simulink model "SSB_10"  (R2018a)
settings: Solver=VariableStepAuto  StartTime=0.0  StopTime=10.0  MaxStep=0.001  RelTol=1e-3
undefined symbols (not defined in the file or in its folder): magnitude
libraries: dspstat3 x2, dsparch4 x1, commrandsrc3 x1, commanapbnd3 x1
settings Model: Creator=sdf  LastModifiedBy=sdf

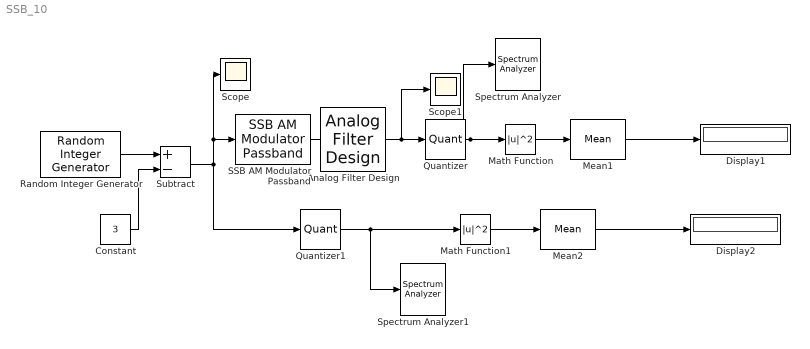
== system SSB_10 ==
  Analog Filter Design : dsparch4/Analog Filter Design  method=Butterworth  filttype=Lowpass  N=8  Wlo=2*pi*300  Whi=80  Rp=2  Rs=40
  Constant : Constant  Value=3
  Display1 : Display
  Display2 : Display
  Math Function : Math  Operator=magnitude^2  SaturateOnIntegerOverflow=on
  Math Function1 : Math  Operator=magnitude^2  SaturateOnIntegerOverflow=on
  Mean1 : dspstat3/Mean  run=on  InputProcessing=Columns as channels (frame based)  reset_popup=None  directionMode=Each column  dimension=1  roiEnable=off  roiType=Rectangles  roiPortion=Entire ROI  roiOutput=Individual statistics for each ROI  roiFlag=off  roundingMode=Floor  overflowMode=off  outputDataTypeStr=Inherit: Same as accumulator  outputMin=[]  outputMax=[]  outputLastDataTypeStr=Inherit: Same as accumulator
  Mean2 : dspstat3/Mean  run=on  InputProcessing=Columns as channels (frame based)  reset_popup=None  directionMode=Each column  dimension=1  roiEnable=off  roiType=Rectangles  roiPortion=Entire ROI  roiOutput=Individual statistics for each ROI  roiFlag=off  roundingMode=Floor  overflowMode=off  outputDataTypeStr=Inherit: Same as accumulator  outputMin=[]  outputMax=[]  outputLastDataTypeStr=Inherit: Same as accumulator
  Quantizer : Quantizer  QuantizationInterval=0.001  LinearizeAsGain=off
  Quantizer1 : Quantizer  QuantizationInterval=0.001  LinearizeAsGain=off
  Random Integer Generator : commrandsrc3/Random Integer Generator  SetSize=7  SeedSource=Parameter  Seed=1234  SampleTime=1/2  SamplesPerFrame=10  OutputDataType=double  SimulateUsing=Interpreted execution
  SSB AM Modulator Passband : commanapbnd3/SSB AM Modulator Passband  Fc=300  Ph=0  Sd=Upper  Ho=100
      settings: SourceProductName=Communications System Toolbox  SourceProductBaseCode=CM
  Scope : Scope
  Scope1 : Scope
  Spectrum Analyzer : SpectrumAnalyzer
  Spectrum Analyzer1 : SpectrumAnalyzer
  Subtract : Sum  Inputs=+-
  wires:
  Random Integer Generator/1 -> Subtract/1
  Constant/1 -> Subtract/2
  Subtract/1 -> Scope/1, SSB AM Modulator Passband/1, Quantizer1/1
  SSB AM Modulator Passband/1 -> Scope1/1, Quantizer/1
  Quantizer1/1 -> Math Function1/1, Spectrum Analyzer1/1
  Quantizer/1 -> Math Function/1, Spectrum Analyzer/1
  Math Function/1 -> Mean1/1
  Mean1/1 -> Display1/1
  Mean2/1 -> Display2/1
  Math Function1/1 -> Mean2/1
